simulink model "Model_14Bus_Microgrid_R2017b"  (R2017b)
settings: Solver=ode23tb  StartTime=0.0  StopTime=0.35  MaxStep=1e-2  RelTol=1e-3
InitFcn:
  | Set_parameters_R2018
StopFcn:
  | Save_Data;
  | Graphics;
values from neighbouring files (symbols this model uses):
  Clink = Ceq*2    (= 0.217013888889)    [Set_parameters_R2017b.m]    (also in Set_parameters_R2018.m)
  dis1 = 0.15    [Set_parameters_R2017b.m]    (also in Set_parameters_R2018.m)
  dis10 = 6    [Set_parameters_R2017b.m]    (also in Set_parameters_R2018.m)
  dis11 = 3    [Set_parameters_R2017b.m]    (also in Set_parameters_R2018.m)
  dis12 = 6    [Set_parameters_R2017b.m]    (also in Set_parameters_R2018.m)
  dis13 = 3    [Set_parameters_R2017b.m]    (also in Set_parameters_R2018.m)
  dis14 = 2    [Set_parameters_R2017b.m]    (also in Set_parameters_R2018.m)
  dis2 = 0.2    [Set_parameters_R2017b.m]    (also in Set_parameters_R2018.m)
  dis3 = 0.15    [Set_parameters_R2017b.m]    (also in Set_parameters_R2018.m)
  dis4 = 0.4    [Set_parameters_R2017b.m]    (also in Set_parameters_R2018.m)
  dis5 = 0.4    [Set_parameters_R2017b.m]    (also in Set_parameters_R2018.m)
  dis6 = 0.4    [Set_parameters_R2017b.m]    (also in Set_parameters_R2018.m)
  dis7 = 0.1    [Set_parameters_R2017b.m]    (also in Set_parameters_R2018.m)
  dis8 = 2    [Set_parameters_R2017b.m]    (also in Set_parameters_R2018.m)
  dis9 = 6    [Set_parameters_R2017b.m]    (also in Set_parameters_R2018.m)
  Fc = 33 * Fnom    (= 1980)    [Set_parameters_R2017b.m]    (also in Set_parameters_R2018.m)
  Fnom = 60    [Main_DC_MG.m]    (also in Set_parameters_R2017b.m; Set_parameters_R2018.m)
  Increment_MPPT = 0.01    [Set_parameters_R2017b.m]    (also in Set_parameters_R2018.m)
  Ki_Ireg = 20    [Set_parameters_R2017b.m]    (also in Set_parameters_R2018.m)
  Ki_VDCreg = 400    [Set_parameters_R2017b.m]    (also in Set_parameters_R2018.m)
  Kp_Ireg = 0.3    [Set_parameters_R2017b.m]    (also in Set_parameters_R2018.m)
  Kp_VDCreg = 2    [Set_parameters_R2017b.m]    (also in Set_parameters_R2018.m)
  LimitL_Ireg = -1.5    [Set_parameters_R2017b.m]    (also in Set_parameters_R2018.m)
  LimitL_VDCreg = -1.5    [Set_parameters_R2017b.m]    (also in Set_parameters_R2018.m)
  Limits_MPPT = [ 583 357 ]    [Set_parameters_R2017b.m]    (also in Set_parameters_R2018.m)
  LimitU_Ireg = 1.5    [Set_parameters_R2017b.m]    (also in Set_parameters_R2018.m)
  LimitU_VDCreg = 1.5    [Set_parameters_R2017b.m]    (also in Set_parameters_R2018.m)
  P_Load_2 = S_Load_2* PF_Load_2    (= 36000)    [Set_parameters_R2017b.m]    (also in Set_parameters_R2018.m)
  P_Load_3 = S_Load_3* PF_Load_3    (= 25500)    [Set_parameters_R2017b.m]    (also in Set_parameters_R2018.m)
  Pnom = 1e6    (= 1000000)    [Set_parameters_R2017b.m]    (also in Set_parameters_R2018.m)
  Pnom_T1 = 1.5e6    (= 1500000)    [Set_parameters_R2017b.m]    (also in Set_parameters_R2018.m)
  Pnom_T2 = 1.5e6    (= 1500000)    [Set_parameters_R2017b.m]    (also in Set_parameters_R2018.m)
  Pnom_T3 = 4e6    (= 4000000)    [Set_parameters_R2017b.m]    (also in Set_parameters_R2018.m)
  Pnom_xfo = Pnom    (= 1000000)    [Set_parameters_R2017b.m]    (also in Set_parameters_R2018.m)
  Ql_Load_2 = S_Load_2 * sin(acos(PF_Load_2))    [Set_parameters_R2017b.m]    (also in Set_parameters_R2018.m)
  Ql_Load_3 = S_Load_3 * sin(acos(PF_Load_3))    [Set_parameters_R2017b.m]    (also in Set_parameters_R2018.m)
  R_Load_9 = (Vnom_prim * 1.35)^2 / P_Load_9    (= 1084.6153125)    [Set_parameters_R2017b.m]    (also in Set_parameters_R2018.m)
  R_Load_DC = Vnom_DC^2/ P_Load_DC    (= 45)    [Main_DC_MG.m]    (also in Set_parameters_R2017b.m; Set_parameters_R2018.m)
  Rl = 0.394    [Set_parameters_R2017b.m]    (also in Set_parameters_R2018.m)
  Rls = 0.198    [Set_parameters_R2017b.m]    (also in Set_parameters_R2018.m)
  Ts = Ts_Power    (= 5.05050505051e-06)    [Main_DC_MG.m]    (also in Set_parameters_R2017b.m; Set_parameters_R2018.m)
  Ts_Control = 10*Ts_Power    (= 5.05050505051e-05)    [Main_DC_MG.m]    (also in Set_parameters_R2017b.m; Set_parameters_R2018.m)
  Ts_Power = 1/(33*Fnom)/100    (= 5.05050505051e-06)    [Main_DC_MG.m]    (also in Set_parameters_R2017b.m; Set_parameters_R2018.m)
  V1_LL_T3 = 69e3    (= 69000)    [Set_parameters_R2017b.m]    (also in Set_parameters_R2018.m)
  Vf = 0    [Set_parameters_R2017b.m]    (also in Set_parameters_R2018.m)
  Vfd = 0    [Set_parameters_R2017b.m]    (also in Set_parameters_R2018.m)
  Vnom_DC = 300    [Main_DC_MG.m]    (also in Set_parameters_R2017b.m; Set_parameters_R2018.m)
  Vnom_dc = 480    [Set_parameters_R2017b.m]    (also in Set_parameters_R2018.m)
  Vnom_Diesel = 2.4e3    (= 2400)    [Set_parameters_R2017b.m]    (also in Set_parameters_R2018.m)
  Vnom_prim = 13.8e3    (= 13800)    [Set_parameters_R2017b.m]    (also in Set_parameters_R2018.m)
  Vnom_sec = 220    [Set_parameters_R2017b.m]    (also in Set_parameters_R2018.m)
  Vnom_ter_AC_DC = 150    [Set_parameters_R2017b.m]    (also in Set_parameters_R2018.m)
  Xl = 0.1168    [Set_parameters_R2017b.m]    (also in Set_parameters_R2018.m)
  Xls = 0.1089    [Set_parameters_R2017b.m]    (also in Set_parameters_R2018.m)
undefined symbols (not defined in the file or in its folder): D1, Delta, Hydride, Ion, Lithium, max_min, Metal, Nickel, RL, RLff, sigbuilder_block
libraries: powerlib x202, powerlib_meascontrol x152, simulink x14, powerlib_extras x14, electricdrivelib x4, re_lib x2
(part 4 of 10)

== system Model_14Bus_Microgrid_R2017b/Bus_AC//DC4 ==
  note: C
  note: B
  note: A
  note: C
  note: Linea - Neutro
  note: B
  note: A
  note: C
  note: B
  note: A
  Conv pu1 : Gain  Gain=sqrt (3) /Vnom_ter_AC_DC  SaturateOnIntegerOverflow=on  OutDataTypeStr=Inherit: Same as input  ParamDataTypeStr=Inherit: Same as input
  Conv pu2 : Gain  Gain=sqrt (3) /Vnom_ter_AC_DC  SaturateOnIntegerOverflow=on  OutDataTypeStr=Inherit: Same as input  ParamDataTypeStr=Inherit: Same as input
  Measurement1 : Scope  NumInputPorts=4
  PLL : Subsystem
  PLL (3ph) : powerlib_meascontrol/PLL/PLL (3ph)  Fmin=45  Par_Init=[0, 60]  ParK=[180, 3200, 1]  TcD=1e-4  MaxRateChangeFreq=12  FilterCutOffFreq=25  Ts=0  AGC=on
      settings: SourceProductName=Simscape Electrical
  Power Factor Block1 : Subsystem  mask(Power Factor Block){Freq=Fnom, Vinit=[0, 0], Iinit=[0, 0], Ts=0}
      mask prompts: Freq "Fundamental frequency (Hz):"; Vinit "Voltage initial input [ Mag, Phase (degrees) ]:"; Iinit "Current initial input [ Mag, Phase (degrees) ]:"; Ts "Sample time:"
      mask help:
      | Power Factor Block developed by Dr Rodney Tan
      | Version 1.01 (Aug 2016)
      |
      | Compute power factor and phase angle of AC circuit voltage-current pair at fundamental frequency.
      |
      | The computation is based on Power block and Complex number function block.
      |
      | For the first cycle of simulation, the outputs are held constant to the powers computed for the Voltage initial input and Current initial input parameters.
      mask Help:
      | <b>Fundamental Frequency (Hz)</b>
      | Specify the measurement fundamental frequency, in hertz, of the input signal.
      | 
      | <b>Voltage initial input [ Mag, Phase (degrees) ]</b>
      | Specify the voltage initial magnitude and phase to set a constant output for the first cycle of simulation.
      | 
      | <b>Current initial input [ Mag, Phase (degrees) ]</b>
      | Specify the current initial magnitude and phase to set a constant output for the first cycle of simulation.
      | 
      | <b>Sample Time</b>
      | Specify the sample time of the block, in seconds. Set to 0 to implement a continuous block.
      mask TypeOptions Freq: Power/Freq
      mask TypeOptions Vinit: Power/Vinit
      mask TypeOptions Iinit: Power/Iinit
      mask TypeOptions Ts: Power/Ts
  Power Factor1 : Display
  Scope : Scope
  Scope1 : Scope
  Scope2 : Scope
  THD : powerlib_meascontrol/Measurements/THD  Freq=60  Ts=Ts_Power
      settings: SourceProductName=Simscape Electrical
  THD (% and signal) : Scope  NumInputPorts=2
  THD (%) : Display
      settings: Format=bank
  Terminator : Terminator
  Vabc pu1 : Scope
  frecuency (Hz) : Display
  to % : Gain  Gain=100  SampleTime=Ts_Power
  ángulo de V (%)1 : Display
      settings: Format=bank
  wires:
  [Iabc_B1_busDC1] -> Power Factor Block1/2(Iabc)
  THD/1 -> to %/1
  to %/1 -> THD (%)/1, THD (% and signal)/2  "THD (%)"
  Power Factor Block1/4(Iabc y Iabc (rms)) -> Measurement1/4
  Power Factor Block1/1(Pabc) -> Measurement1/1
  Conv pu1/1 -> Vabc pu1/1
  Power Factor Block1/5("PFabc ") -> Scope1/1, Power Factor1/1
  Power Factor Block1/2(Qabc) -> Measurement1/2
  Power Factor Block1/3(Vabc y Vabc (rms)) -> Conv pu1/1, Measurement1/3
  PLL/1(delta_abc) -> Scope/1, ángulo de V (%)1/1
  Conv pu2/1 -> PLL/1(Vabc_LN_pu)
  PLL (3ph)/2 -> Terminator/1
  [Vabc_B1_busDC1] -> PLL (3ph)/1, Conv pu2/1, THD/1, THD (% and signal)/1, Power Factor Block1/1(Vabc)  "Vabc"
  PLL (3ph)/1 -> Scope2/1, frecuency (Hz)/1

== system Model_14Bus_Microgrid_R2017b/Bus_AC//DC5 ==
  note: C
  note: B
  note: A
  note: C
  note: Linea - Neutro
  note: B
  note: A
  note: B
  note: C
  note: A
  Conv pu1 : Gain  Gain=sqrt (3) /Vnom_ter_AC_DC  SaturateOnIntegerOverflow=on  OutDataTypeStr=Inherit: Same as input  ParamDataTypeStr=Inherit: Same as input
  Conv pu2 : Gain  Gain=sqrt (3) /Vnom_ter_AC_DC  SaturateOnIntegerOverflow=on  OutDataTypeStr=Inherit: Same as input  ParamDataTypeStr=Inherit: Same as input
  Measurement1 : Scope  NumInputPorts=4
  PLL : Subsystem
  PLL (3ph) : powerlib_meascontrol/PLL/PLL (3ph)  Fmin=45  Par_Init=[0, 60]  ParK=[180, 3200, 1]  TcD=1e-4  MaxRateChangeFreq=12  FilterCutOffFreq=25  Ts=0  AGC=on
      settings: SourceProductName=Simscape Electrical
  Power Factor Block1 : Subsystem  mask(Power Factor Block){Freq=Fnom, Vinit=[0, 0], Iinit=[0, 0], Ts=0}
      mask prompts: Freq "Fundamental frequency (Hz):"; Vinit "Voltage initial input [ Mag, Phase (degrees) ]:"; Iinit "Current initial input [ Mag, Phase (degrees) ]:"; Ts "Sample time:"
      mask help:
      | Power Factor Block developed by Dr Rodney Tan
      | Version 1.01 (Aug 2016)
      |
      | Compute power factor and phase angle of AC circuit voltage-current pair at fundamental frequency.
      |
      | The computation is based on Power block and Complex number function block.
      |
      | For the first cycle of simulation, the outputs are held constant to the powers computed for the Voltage initial input and Current initial input parameters.
      mask Help:
      | <b>Fundamental Frequency (Hz)</b>
      | Specify the measurement fundamental frequency, in hertz, of the input signal.
      | 
      | <b>Voltage initial input [ Mag, Phase (degrees) ]</b>
      | Specify the voltage initial magnitude and phase to set a constant output for the first cycle of simulation.
      | 
      | <b>Current initial input [ Mag, Phase (degrees) ]</b>
      | Specify the current initial magnitude and phase to set a constant output for the first cycle of simulation.
      | 
      | <b>Sample Time</b>
      | Specify the sample time of the block, in seconds. Set to 0 to implement a continuous block.
      mask TypeOptions Freq: Power/Freq
      mask TypeOptions Vinit: Power/Vinit
      mask TypeOptions Iinit: Power/Iinit
      mask TypeOptions Ts: Power/Ts
  Power Factor1 : Display
  Scope : Scope
  Scope1 : Scope
  Scope2 : Scope
  THD : powerlib_meascontrol/Measurements/THD  Freq=60  Ts=Ts_Power
      settings: SourceProductName=Simscape Electrical
  THD (% and signal) : Scope  NumInputPorts=2
  THD (%) : Display
      settings: Format=bank
  Terminator : Terminator
  Vabc pu1 : Scope
  frecuency (Hz) : Display
  to % : Gain  Gain=100  SampleTime=Ts_Power
  ángulo de V (%)1 : Display
      settings: Format=bank
  wires:
  [Iabc_B1_busDC2] -> Power Factor Block1/2(Iabc)
  THD/1 -> to %/1
  to %/1 -> THD (%)/1, THD (% and signal)/2  "THD (%)"
  Power Factor Block1/4(Iabc y Iabc (rms)) -> Measurement1/4
  Power Factor Block1/1(Pabc) -> Measurement1/1
  Conv pu1/1 -> Vabc pu1/1
  Power Factor Block1/5("PFabc ") -> Scope1/1, Power Factor1/1
  Power Factor Block1/2(Qabc) -> Measurement1/2
  Power Factor Block1/3(Vabc y Vabc (rms)) -> Conv pu1/1, Measurement1/3
  Conv pu2/1 -> PLL/1(Vabc_LN_pu)
  PLL/1(delta_abc) -> Scope/1, ángulo de V (%)1/1
  PLL (3ph)/2 -> Terminator/1
  [Vabc_B1_busDC2] -> Power Factor Block1/1(Vabc), PLL (3ph)/1, Conv pu2/1, THD/1, THD (% and signal)/1  "Vabc"
  PLL (3ph)/1 -> Scope2/1, frecuency (Hz)/1

== system Model_14Bus_Microgrid_R2017b/Bus_slack  ==
  note: C
  note: B
  note: A
  note: C
  note: Linea - Neutro
  note: B
  note: A
  note: A
  note: B
  note: C
  Conv pu1 : Gain  Gain=sqrt (3) /Vnom_prim  SaturateOnIntegerOverflow=on  OutDataTypeStr=Inherit: Same as input  ParamDataTypeStr=Inherit: Same as input
  Conv pu2 : Gain  Gain=sqrt (3) /Vnom_prim  SaturateOnIntegerOverflow=on  OutDataTypeStr=Inherit: Same as input  ParamDataTypeStr=Inherit: Same as input
  Measurement1 : Scope  NumInputPorts=4
  PLL : Subsystem
  PLL (3ph) : powerlib_meascontrol/PLL/PLL (3ph)  Fmin=45  Par_Init=[0, 60]  ParK=[180, 3200, 1]  TcD=1e-4  MaxRateChangeFreq=12  FilterCutOffFreq=25  Ts=0  AGC=on
      settings: SourceProductName=Simscape Electrical
  Power Factor Block1 : Subsystem  mask(Power Factor Block){Freq=Fnom, Vinit=[0, 0], Iinit=[0, 0], Ts=0}
      mask prompts: Freq "Fundamental frequency (Hz):"; Vinit "Voltage initial input [ Mag, Phase (degrees) ]:"; Iinit "Current initial input [ Mag, Phase (degrees) ]:"; Ts "Sample time:"
      mask help:
      | Power Factor Block developed by Dr Rodney Tan
      | Version 1.01 (Aug 2016)
      |
      | Compute power factor and phase angle of AC circuit voltage-current pair at fundamental frequency.
      |
      | The computation is based on Power block and Complex number function block.
      |
      | For the first cycle of simulation, the outputs are held constant to the powers computed for the Voltage initial input and Current initial input parameters.
      mask Help:
      | <b>Fundamental Frequency (Hz)</b>
      | Specify the measurement fundamental frequency, in hertz, of the input signal.
      | 
      | <b>Voltage initial input [ Mag, Phase (degrees) ]</b>
      | Specify the voltage initial magnitude and phase to set a constant output for the first cycle of simulation.
      | 
      | <b>Current initial input [ Mag, Phase (degrees) ]</b>
      | Specify the current initial magnitude and phase to set a constant output for the first cycle of simulation.
      | 
      | <b>Sample Time</b>
      | Specify the sample time of the block, in seconds. Set to 0 to implement a continuous block.
      mask TypeOptions Freq: Power/Freq
      mask TypeOptions Vinit: Power/Vinit
      mask TypeOptions Iinit: Power/Iinit
      mask TypeOptions Ts: Power/Ts
  Power Factor1 : Display
  Scope : Scope
  Scope2 : Scope
  THD : powerlib_meascontrol/Measurements/THD  Freq=60  Ts=Ts_Power
      settings: SourceProductName=Simscape Electrical
  THD (% and signal) : Scope  NumInputPorts=2
  THD (%) : Display
      settings: Format=bank
  Terminator : Terminator
  Vabc pu1 : Scope
  frecuency (Hz) : Display
  to % : Gain  Gain=100  SampleTime=Ts_Power
  ángulo de V (%)1 : Display
      settings: Format=bank
  tag scope: PFabc_Bus13=global, THDv_abc_Bus13=global, delta_abc_Bus13=global
  wires:
  [Iabc_Sec] -> Power Factor Block1/2(Iabc)  "Signal Iabc"
  THD/1 -> to %/1
  Power Factor Block1/4(Iabc y Iabc (rms)) -> Measurement1/4
  Power Factor Block1/1(Pabc) -> Measurement1/1
  Conv pu1/1 -> Vabc pu1/1
  Power Factor Block1/2(Qabc) -> Measurement1/2
  Power Factor Block1/3(Vabc y Vabc (rms)) -> Conv pu1/1, Measurement1/3
  to %/1 -> [THDv_abc_Bus13], THD (%)/1, THD (% and signal)/2  "THD (%)"
  Power Factor Block1/5("PFabc ") -> [PFabc_Bus13], Power Factor1/1
  Conv pu2/1 -> PLL/1(Vabc_LN_pu)
  PLL/1(delta_abc) -> [delta_abc_Bus13], Scope/1, ángulo de V (%)1/1
  [Vabc_Sec] -> Power Factor Block1/1(Vabc), THD/1, THD (% and signal)/1, PLL (3ph)/1, Conv pu2/1  "Vabc"
  PLL (3ph)/2 -> Terminator/1
  PLL (3ph)/1 -> Scope2/1, frecuency (Hz)/1

== system Model_14Bus_Microgrid_R2017b/Control measurement ==
  note: VL-L rms
  Bus Creator : BusCreator  Inputs=4
  VL-L : Scope  NumInputPorts=2
  Vph_rms : Scope
  m1 : Scope
  measurement : Subsystem
  "                                          C" : PMIOPort  Side=Left
  "                                          B" : PMIOPort  Port=2  Side=Left
  "                                          A" : PMIOPort  Port=3  Side=Left
  "              Out1" : Outport
  wires:
  measurement/2(VL-L) -> VL-L/1, Bus Creator/2
  measurement/3(VL-L_rms) -> VL-L/2, Bus Creator/3
  measurement/4(Vph_rms) -> Vph_rms/1, Bus Creator/4
  measurement/1(Vph) -> m1/1, Bus Creator/1
  Bus Creator/1 -> "              Out1"/1
  connections:
  "                                          A"/RConn1 -- measurement/LConn1
  "                                          B"/RConn1 -- measurement/LConn2
  "                                          C"/RConn1 -- measurement/LConn3

== system Model_14Bus_Microgrid_R2017b/Control measurement2 ==
  note: VL-L rms_3
  Bus Creator : BusCreator  Inputs=4
  VL-L_3 : Scope  NumInputPorts=2
  Vph_rms_3 : Scope
  m1_3 : Scope
  measurement2 : Subsystem
  "                                          C" : PMIOPort  Side=Left
  "                                          B" : PMIOPort  Port=2  Side=Left
  "                                          A" : PMIOPort  Port=3  Side=Left
  "              Out1" : Outport
  wires:
  measurement2/2(VL-L) -> VL-L_3/1, Bus Creator/2
  measurement2/3(VL-L_rms) -> VL-L_3/2, Bus Creator/3
  measurement2/4(Vph_rms) -> Vph_rms_3/1, Bus Creator/4
  measurement2/1(Vph) -> m1_3/1, Bus Creator/1
  Bus Creator/1 -> "              Out1"/1
  connections:
  "                                          A"/RConn1 -- measurement2/LConn1
  "                                          B"/RConn1 -- measurement2/LConn2
  "                                          C"/RConn1 -- measurement2/LConn3

== system Model_14Bus_Microgrid_R2017b/DATA  ADQUISITION ==
  note: Transformer (T1)
  note: Paper: "Hybrid AC/DC Microgrid test system simulation: Grid-connected mode"
  Delta_abc : Subsystem
  PF_abc : Subsystem
  P_abc : Subsystem
  Power_Losses_abc : Subsystem
  Q_abc : Subsystem
  RMS1 : powerlib_meascontrol/Measurements/RMS  TrueRMS=on  Freq=60  RMSInit=0  Ts=0
      settings: SourceProductName=Simscape Electrical
  RMS2 : powerlib_meascontrol/Measurements/RMS  TrueRMS=on  Freq=60  RMSInit=0  Ts=0
      settings: SourceProductName=Simscape Electrical
  THDv_abc : Subsystem
  VoltageLL_pu_abc : Subsystem
  scope 11 : Scope
  scope 12 : Scope
  wires:
  [Vabc_Sec_pu] -> RMS1/1
  RMS1/1 -> scope 11/1
  RMS2/1 -> scope 12/1
  [Vabc_Prim_pu] -> RMS2/1  "Signal Vabc"

== system Model_14Bus_Microgrid_R2017b/Diesel_ 3MVA ==
  note: Diesel generator 2
  2.4kV  50MVA : powerlib/Elements/Three-Phase Series RLC Branch  LConnTagsString=A|B|C  RConnTagsString=A|B|C  BranchType=RL  Resistance=2.4e3^2/50e6/10  Inductance=2.4e3^2/50e6/(2*pi*60)  Capacitance=1.0  Measurements=None
      settings: SourceProductName=Simscape Electrical
  Ground1 : powerlib/Elements/Ground  LConnTagsString=a
      settings: SourceProductName=Simscape Electrical
  Programmable Voltage Source1 : powerlib/Electrical Sources/Three-Phase Programmable Voltage Source  PositiveSequence="[Vnom_Diesel*0.9848 -60  Fnom]"  VariationEntity=None  VariationType=Table of time-amplitude pairs  VariationTypeAlt=Step  VariationStep=-0.3  VariationRate=0.5  VariationMagnitude=0.4  VariationFrequency=2  VariationTiming=[0.1 1.2]  VariationPhaseA=off  Amplitudes=[1]  TimeValues=[0]  HarmonicGeneration=off  HarmonicA=[3 0.2 -25 0]  HarmonicB="[2 0.15  35 2]"  Timing="[0.1  0.6]"  BusType=PV  Pref=Pgen_Diesel  Qref=0  Qmin=-inf  Qmax=inf
      settings: SourceProductName=Simscape Electrical
  a1 : PMIOPort  Tag=PMCPort  Side=Left
  b1 : PMIOPort  Tag=PMCPort  Port=2  Side=Left
  c1 : PMIOPort  Tag=PMCPort  Port=3  Side=Left
  connections:
  Programmable Voltage Source1/RConn3 -- 2.4kV  50MVA/LConn3
  Ground1/LConn1 -- Programmable Voltage Source1/LConn1
  Programmable Voltage Source1/RConn2 -- 2.4kV  50MVA/LConn2
  2.4kV  50MVA/LConn1 -- Programmable Voltage Source1/RConn1
  b1/RConn1 -- 2.4kV  50MVA/RConn2
  a1/RConn1 -- 2.4kV  50MVA/RConn1
  c1/RConn1 -- 2.4kV  50MVA/RConn3

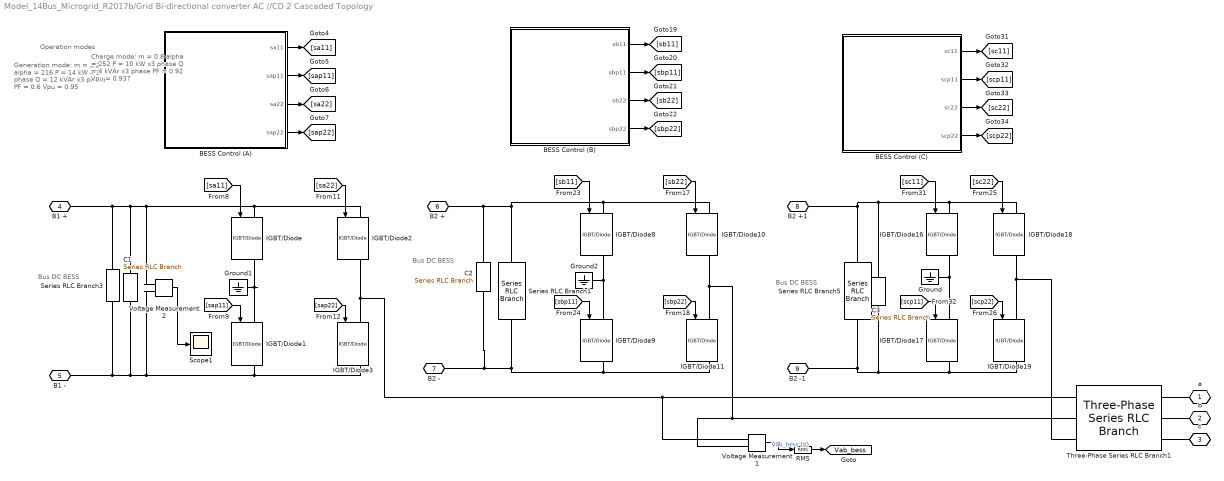
== system Model_14Bus_Microgrid_R2017b/Grid Bi-directional converter AC //CD 2 Cascaded Topology ==
  note: Operation modes
  note: Generation mode:
      |
      | m = 1.2
      | alpha = 216
      |
      | P = 14 kW x 3 phase
      | Q = 12 kVAr x3 phase
      | PF = 0.6
      | Vpu = 0.95
  note: Bus DC BESS
  note: Bus DC BESS
  note: Bus DC BESS
  note: Charge mode:
      |
      | m = 0.8
      | alpha = 252
      |
      | P = 10 kW x3 phase
      | Q = 4 kVAr x3 phase
      | PF = 0.92
      | Vpu = 0.937
  BESS Control (A) : Subsystem
      mask Display: image('Icons\FPGA.png');
  BESS Control (B) : Subsystem
      mask Display: image('Icons\FPGA.png');
  BESS Control (C) : Subsystem
      mask Display: image('Icons\FPGA.png');
  C1 : powerlib/Elements/Series RLC Branch  LConnTagsString=__new0  RConnTagsString=__new0  BranchType=C  Resistance=22.5  Inductance=1e-3  SetiL0=off  InitialCurrent=0  Capacitance=10e-3  Setx0=off  InitialVoltage=0  Measurements=None
      settings: SourceProductName=Simscape Electrical
  C2 : powerlib/Elements/Series RLC Branch  LConnTagsString=__new0  RConnTagsString=__new0  BranchType=C  Resistance=22.5  Inductance=1e-3  SetiL0=off  InitialCurrent=0  Capacitance=10e-3  Setx0=off  InitialVoltage=0  Measurements=None
      settings: SourceProductName=Simscape Electrical
  C3 : powerlib/Elements/Series RLC Branch  LConnTagsString=__new0  RConnTagsString=__new0  BranchType=C  Resistance=22.5  Inductance=1e-3  SetiL0=off  InitialCurrent=0  Capacitance=10e-3  Setx0=off  InitialVoltage=0  Measurements=None
      settings: SourceProductName=Simscape Electrical
  Ground : powerlib/Elements/Ground  LConnTagsString=a
      settings: SourceProductName=Simscape Electrical
  Ground1 : powerlib/Elements/Ground  LConnTagsString=a
      settings: SourceProductName=Simscape Electrical
  Ground2 : powerlib/Elements/Ground  LConnTagsString=a
      settings: SourceProductName=Simscape Electrical
  IGBT/Diode{,1..3,8..11,16..19} (12 alike) : powerlib/Power Electronics/IGBT//Diode  Ron=1e-3  Rs=1e5  Cs=inf  Measurements=on
      settings: SourceProductName=Simscape Electrical
  RMS : powerlib_meascontrol/Measurements/RMS  TrueRMS=off  Freq=60  RMSInit=1  Ts=0
      settings: SourceProductName=Simscape Electrical
  Scope1 : Scope
  Series RLC Branch1 : powerlib/Elements/Series RLC Branch  LConnTagsString=__new0  RConnTagsString=__new0  BranchType=R  Resistance=1e9  Inductance=1e-3  SetiL0=off  InitialCurrent=0  Capacitance=1e-6  Setx0=off  InitialVoltage=0  Measurements=None
      settings: SourceProductName=Simscape Electrical
  Series RLC Branch3 : powerlib/Elements/Series RLC Branch  LConnTagsString=__new0  RConnTagsString=__new0  BranchType=R  Resistance=1e9  Inductance=1e-3  SetiL0=off  InitialCurrent=0  Capacitance=1e-6  Setx0=off  InitialVoltage=0  Measurements=None
      settings: SourceProductName=Simscape Electrical
  Series RLC Branch5 : powerlib/Elements/Series RLC Branch  LConnTagsString=__new0  RConnTagsString=__new0  BranchType=R  Resistance=1e9  Inductance=1e-3  SetiL0=off  InitialCurrent=0  Capacitance=1e-6  Setx0=off  InitialVoltage=0  Measurements=None
      settings: SourceProductName=Simscape Electrical
  Three-Phase Series RLC Branch1 : powerlib/Elements/Three-Phase Series RLC Branch  LConnTagsString=A|B|C  RConnTagsString=A|B|C  BranchType=RL  Resistance=1  Inductance=1.2e-2  Capacitance=15.5e-5  Measurements=None
      settings: SourceProductName=Simscape Electrical
  Voltage Measurement1 : powerlib/Measurements/Voltage Measurement  PhasorSimulation=off  OutputType=Complex  PSBequivalent=0
      settings: SourceProductName=Simscape Electrical
  Voltage Measurement2 : powerlib/Measurements/Voltage Measurement  PhasorSimulation=off  OutputType=Complex  PSBequivalent=0
      settings: SourceProductName=Simscape Electrical
  "a " : PMIOPort  Tag=PMCPort  Side=Left
  b : PMIOPort  Tag=PMCPort  Port=2  Side=Left
  c : PMIOPort  Tag=PMCPort  Port=3  Side=Left
  B1 + : PMIOPort  Port=4  Side=Right
  B1 - : PMIOPort  Port=5  Side=Right
  B2 + : PMIOPort  Port=6  Side=Right
  B2 - : PMIOPort  Port=7  Side=Right
  B2 +1 : PMIOPort  Port=8  Side=Right
  B2 -1 : PMIOPort  Port=9  Side=Right
  tag scope: Vab_bess=global
  wires:
  [sa11] -> IGBT/Diode/1
  [sap11] -> IGBT/Diode1/1
  [sa22] -> IGBT/Diode2/1
  [sap22] -> IGBT/Diode3/1
  [sb11] -> IGBT/Diode8/1
  [sbp11] -> IGBT/Diode9/1
  [sb22] -> IGBT/Diode10/1
  [sbp22] -> IGBT/Diode11/1
  [sc11] -> IGBT/Diode16/1
  [scp11] -> IGBT/Diode17/1
  [sc22] -> IGBT/Diode18/1
  [scp22] -> IGBT/Diode19/1
  Voltage Measurement1/1 -> RMS/1  "Vab_bess (V)"
  RMS/1 -> [Vab_bess]
  Voltage Measurement2/1 -> Scope1/1
  BESS Control (A)/1(sa11) -> [sa11]
  BESS Control (A)/2(sap11) -> [sap11]
  BESS Control (A)/3(sa22) -> [sa22]
  BESS Control (A)/4(sap22) -> [sap22]
  BESS Control (B)/1(sb11) -> [sb11]
  BESS Control (B)/2(sbp11) -> [sbp11]
  BESS Control (B)/3(sb22) -> [sb22]
  BESS Control (B)/4(sbp22) -> [sbp22]
  BESS Control (C)/1(sc11) -> [sc11]
  BESS Control (C)/2(scp11) -> [scp11]
  BESS Control (C)/3(sc22) -> [sc22]
  BESS Control (C)/4(scp22) -> [scp22]
  connections:
  IGBT/Diode1/RConn1 -- IGBT/Diode3/RConn1 -- C1/RConn1 -- Series RLC Branch3/RConn1 -- B1 -/RConn1 -- Voltage Measurement2/LConn2
  Series RLC Branch1/RConn1 -- C2/RConn1 -- B2 -/RConn1 -- IGBT/Diode9/RConn1 -- IGBT/Diode11/RConn1
  IGBT/Diode11/LConn1 -- Voltage Measurement1/LConn2 -- Three-Phase Series RLC Branch1/LConn2 -- IGBT/Diode10/RConn1
  Series RLC Branch5/RConn1 -- B2 -1/RConn1 -- C3/RConn1 -- IGBT/Diode19/RConn1 -- IGBT/Diode17/RConn1
  IGBT/Diode19/LConn1 -- Three-Phase Series RLC Branch1/LConn3 -- IGBT/Diode18/RConn1
  IGBT/Diode/LConn1 -- IGBT/Diode2/LConn1 -- Voltage Measurement2/LConn1 -- C1/LConn1 -- B1 +/RConn1 -- Series RLC Branch3/LConn1
  Voltage Measurement1/LConn1 -- IGBT/Diode2/RConn1 -- IGBT/Diode3/LConn1 -- Three-Phase Series RLC Branch1/LConn1
  IGBT/Diode8/LConn1 -- C2/LConn1 -- B2 +/RConn1 -- Series RLC Branch1/LConn1 -- IGBT/Diode10/LConn1
  IGBT/Diode16/LConn1 -- C3/LConn1 -- Series RLC Branch5/LConn1 -- B2 +1/RConn1 -- IGBT/Diode18/LConn1
  IGBT/Diode1/LConn1 -- Ground1/LConn1 -- IGBT/Diode/RConn1
  IGBT/Diode9/LConn1 -- Ground2/LConn1 -- IGBT/Diode8/RConn1
  IGBT/Diode16/RConn1 -- Ground/LConn1 -- IGBT/Diode17/LConn1
  "a "/RConn1 -- Three-Phase Series RLC Branch1/RConn1
  b/RConn1 -- Three-Phase Series RLC Branch1/RConn2
  c/RConn1 -- Three-Phase Series RLC Branch1/RConn3

== system Model_14Bus_Microgrid_R2017b/Grid Bi-directional Converter 1.1 300 (DC) // 150 V (AC) P_nom 3kW ==
  note: Bus DC
  note: Bus AC
  note: Inverter mode:
      |
      | m = 1.2
      | alpha = 0
      |
      | P = 1 kW x 3 phase
      | Q = 1 kVAr x3 phase
      | PF = 0.6
      | Vpu = 0.95
  note: Operation modes
  note: Rectif mode:
      |
      | m = 1
      | alpha = 228
      |
      | P = 975 kVA (DC)
  Means : Inport
  C1 : powerlib/Elements/Series RLC Branch  LConnTagsString=__new0  RConnTagsString=__new0  BranchType=C  Resistance=22.5  Inductance=1e-3  SetiL0=off  InitialCurrent=0  Capacitance=1200e-6  Setx0=off  InitialVoltage=150  Measurements=None
      settings: SourceProductName=Simscape Electrical
  Control of Inverter : Subsystem
      mask Display: image('Icons\FPGA.png');
  Ground1 : powerlib/Elements/Ground  LConnTagsString=a
      settings: SourceProductName=Simscape Electrical
  Scope : Scope
  Three-Phase Parallel RLC Branch1 : powerlib/Elements/Three-Phase Parallel RLC Branch  LConnTagsString=A|B|C  RConnTagsString=A|B|C  BranchType=C  Resistance=1  Inductance=1e-3  Capacitance=2.65e-6  Measurements=None
      settings: SourceProductName=Simscape Electrical  SourceProductBaseCode=PS
  Three-Phase Series RLC Branch1 : powerlib/Elements/Three-Phase Series RLC Branch  LConnTagsString=A|B|C  RConnTagsString=A|B|C  BranchType=RL  Resistance=2  Inductance=1e-2  Capacitance=15.5e-5  Measurements=None
      settings: SourceProductName=Simscape Electrical
  Universal Bridge1 : powerlib/Power Electronics/Universal Bridge  Arms=3  SnubberResistance=1e5  SnubberCapacitance=inf  Device=MOSFET / Diodes  Ron=1e-3  Lon=0  ForwardVoltages="[  0  0  ]"  ForwardVoltage=0  GTOparameters=[ 10e-6 , 20e-6 ]  IGBTparameters=[ 1e-6 , 2e-6 ]  Measurements=None  Measurements_2=None  converterType=Rectifier
      settings: SourceProductName=Simscape Electrical
  "a " : PMIOPort  Tag=PMCPort  Side=Left
  b : PMIOPort  Tag=PMCPort  Port=2  Side=Left
  c : PMIOPort  Tag=PMCPort  Port=3  Side=Left
  B1 + : PMIOPort  Port=4  Side=Right
  B1 - : PMIOPort  Port=5  Side=Right
  tag scope: Pulse=global
  wires:
  Control of Inverter/1(Pulses) -> Scope/1, [Pulse]
  [Pulse] -> Universal Bridge1/1
  Means/1 -> Control of Inverter/1(Means)
  connections:
  Three-Phase Series RLC Branch1/RConn1 -- Three-Phase Parallel RLC Branch1/LConn1 -- "a "/RConn1
  Three-Phase Parallel RLC Branch1/LConn2 -- Three-Phase Series RLC Branch1/RConn2 -- b/RConn1
  Three-Phase Parallel RLC Branch1/LConn3 -- Three-Phase Series RLC Branch1/RConn3 -- c/RConn1
  Ground1/LConn1 -- Three-Phase Parallel RLC Branch1/RConn3 -- Three-Phase Parallel RLC Branch1/RConn1 -- Three-Phase Parallel RLC Branch1/RConn2
  Universal Bridge1/LConn3 -- Three-Phase Series RLC Branch1/LConn3
  Three-Phase Series RLC Branch1/LConn2 -- Universal Bridge1/LConn2
  Universal Bridge1/LConn1 -- Three-Phase Series RLC Branch1/LConn1
  B1 +/RConn1 -- C1/LConn1 -- Universal Bridge1/RConn1
  B1 -/RConn1 -- C1/RConn1 -- Universal Bridge1/RConn2

== system Model_14Bus_Microgrid_R2017b/Grid Bi-directional Converter 1.2 300 (DC) // 150 V (AC) P_nom 3kW ==
  note: DC Bus
  note: AC Bus
  note: Inverter mode:
      |
      | m = 1.2
      | alpha = 0
      |
      | P = 1 kW x 3 phase
      | Q = 1 kVAr x3 phase
      | PF = 0.6
      | Vpu = 0.95
  note: Rectif mode:
      |
      | NO WORK
  Means2 : Inport
  C1 : powerlib/Elements/Series RLC Branch  LConnTagsString=__new0  RConnTagsString=__new0  BranchType=C  Resistance=22.5  Inductance=1e-3  SetiL0=off  InitialCurrent=0  Capacitance=1200e-6  Setx0=off  InitialVoltage=150  Measurements=None
      settings: SourceProductName=Simscape Electrical
  Control of Inverter : Subsystem
      mask Display: image('Icons\FPGA.png');
  Ground1 : powerlib/Elements/Ground  LConnTagsString=a
      settings: SourceProductName=Simscape Electrical
  Scope : Scope
  Three-Phase Parallel RLC Branch2 : powerlib/Elements/Three-Phase Parallel RLC Branch  LConnTagsString=A|B|C  RConnTagsString=A|B|C  BranchType=C  Resistance=1  Inductance=1e-3  Capacitance=2.65e-6  Measurements=None
      settings: SourceProductName=Simscape Electrical  SourceProductBaseCode=PS
  Three-Phase Series RLC Branch2 : powerlib/Elements/Three-Phase Series RLC Branch  LConnTagsString=A|B|C  RConnTagsString=A|B|C  BranchType=RL  Resistance=2  Inductance=1e-2  Capacitance=15.5e-5  Measurements=None
      settings: SourceProductName=Simscape Electrical
  Universal Bridge2 : powerlib/Power Electronics/Universal Bridge  Arms=3  SnubberResistance=1e5  SnubberCapacitance=inf  Device=MOSFET / Diodes  Ron=1e-3  Lon=0  ForwardVoltages="[  0  0  ]"  ForwardVoltage=0  GTOparameters=[ 10e-6 , 20e-6 ]  IGBTparameters=[ 1e-6 , 2e-6 ]  Measurements=None  Measurements_2=None  converterType=Rectifier
      settings: SourceProductName=Simscape Electrical
  "a " : PMIOPort  Tag=PMCPort  Side=Left
  b : PMIOPort  Tag=PMCPort  Port=2  Side=Left
  c : PMIOPort  Tag=PMCPort  Port=3  Side=Left
  B1 + : PMIOPort  Port=4  Side=Right
  B1 - : PMIOPort  Port=5  Side=Right
  tag scope: Pulse2=global
  wires:
  Control of Inverter/1(Pulses) -> Scope/1, [Pulse2]
  Means2/1 -> Control of Inverter/1(Means2)
  [Pulse2] -> Universal Bridge2/1
  connections:
  Three-Phase Series RLC Branch2/RConn1 -- Three-Phase Parallel RLC Branch2/LConn1 -- "a "/RConn1
  Three-Phase Parallel RLC Branch2/LConn2 -- Three-Phase Series RLC Branch2/RConn2 -- b/RConn1
  Three-Phase Parallel RLC Branch2/LConn3 -- Three-Phase Series RLC Branch2/RConn3 -- c/RConn1
  Ground1/LConn1 -- Three-Phase Parallel RLC Branch2/RConn3 -- Three-Phase Parallel RLC Branch2/RConn1 -- Three-Phase Parallel RLC Branch2/RConn2
  Universal Bridge2/LConn3 -- Three-Phase Series RLC Branch2/LConn3
  Three-Phase Series RLC Branch2/LConn2 -- Universal Bridge2/LConn2
  Universal Bridge2/LConn1 -- Three-Phase Series RLC Branch2/LConn1
  Universal Bridge2/RConn1 -- B1 +/RConn1 -- C1/LConn1
  B1 -/RConn1 -- Universal Bridge2/RConn2 -- C1/RConn1

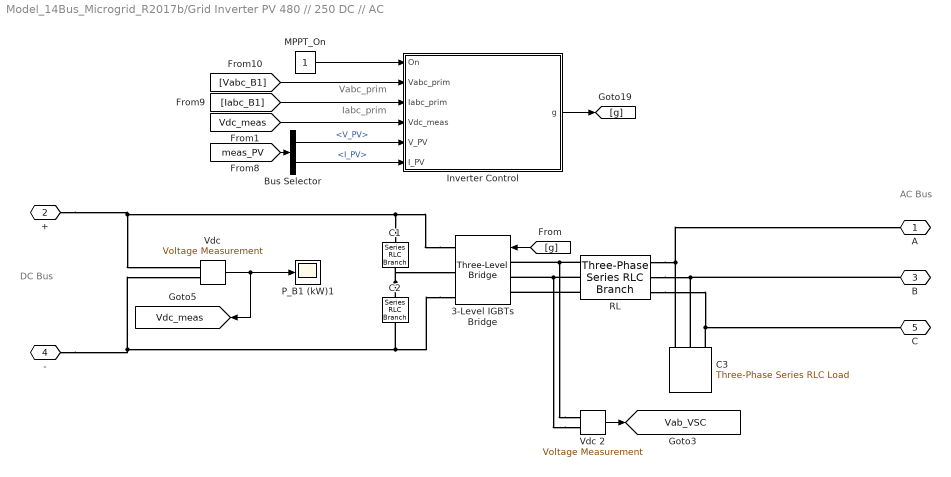
== system Model_14Bus_Microgrid_R2017b/Grid Inverter PV 480 // 250 DC // AC  ==
  note: Iabc_prim
  note: Vabc_prim
  note: AC Bus
  note: DC Bus
  3-Level IGBTs Bridge : powerlib/Power Electronics/Three-Level Bridge  Arms=3  SnubberResistance=Rs  SbubberCapacitance=Cs  Device=IGBT / Diodes  Ron=Ron  ForwardVoltages="[  Vfd  Vf ]"  Measurements=None
      settings: SourceProductName=Simscape Electrical  SourceProductBaseCode=PS
  Bus Selector : BusSelector  OutputSignals=V_PV,I_PV
  C1 : powerlib/Elements/Series RLC Branch  LConnTagsString=__new0  RConnTagsString=__new0  BranchType=C  Resistance=1.0  Inductance=1.0  SetiL0=off  InitialCurrent=0  Capacitance=Clink  Setx0=on  InitialVoltage=Vnom_dc/2  Measurements=None
      settings: SourceProductName=Simscape Electrical
  C2 : powerlib/Elements/Series RLC Branch  LConnTagsString=__new0  RConnTagsString=__new0  BranchType=C  Resistance=1.0  Inductance=1.0  SetiL0=off  InitialCurrent=0  Capacitance=Clink  Setx0=on  InitialVoltage=Vnom_dc/2  Measurements=None
      settings: SourceProductName=Simscape Electrical
  C3 : powerlib/Elements/Three-Phase Series RLC Load  LConnTagsString=A|B|C  Configuration=Delta  NominalVoltage=Vnom_sec  Vabc=[1e3 1e3 1e3]  Vabcp=[1e3 1e3 1e3]  NominalFrequency=Fnom  UnbalancedPower=off  ActivePower=Pc  InductivePower=0  CapacitivePower=Qc  Pabc=[10e3 9e3 11e3]  QLabc=[100 90 110]  QCabc=[100 90 110]  Pabcp=[10e3 9e3 11e3]  QLabcp=[100 90 110]  QCabcp=[100 90 110]  Measurements=None  LoadType=constant Z
      settings: SourceProductName=Simscape Electrical
  Inverter Control : Subsystem  mask(Inverter Control){Pnom=Pnom, Fnom=Fnom, Vnom_prim=Vnom_prim, Vnom_sec=Vnom_sec, Vnom_dc=Vnom_dc, Increment_MPPT=Increment_MPPT, Limits_MPPT=Limits_MPPT, Vdc_ref_Init=Vnom_dc, Kp_VDCreg=Kp_VDCreg, Ki_VDCreg=Ki_VDCreg, Kp_Ireg=Kp_Ireg, Ki_Ireg=Ki_Ireg, RLff=RLff, Fc=Fc, Ts_Control=Ts_Control, Ts_PWMgenerator=Ts_Power}
      mask prompts: Pnom "Power (VA)"; Fnom "Frequency (Hz)"; Vnom_prim "Primary voltage (Vrms LL)"; Vnom_sec "Secondary voltage (Vrms LL)"; Vnom_dc "DC voltage (V)"; Increment_MPPT "Output increment (V)"; Limits_MPPT "Output limits [ Upper  Lower ]"; Vdc_ref_Init "Output initial value (V)"; Kp_VDCreg "Proportional gain"; Ki_VDCreg "Integral gain"; Kp_Ireg "Proportional gain"; Ki_Ireg "Integral gain"; RLff "Feedforward Values [Rff Lff]"; Fc "Carrier frequency (Hz)"; Ts_Control "Control systems"; Ts_PWMgenerator "PWM generator"
      mask help:
      | The main components of the Inverter Control are:
      | 1. PLL & Measurements
      | 2. Maximum Power Point Tracker System (MPPT) using a Perturb & Observe algorithm
      | 3. DC Voltage Regulator
      | 4. Current Regulator
      | 5. PWM Modulator
      mask DialogControl Container4 Prompt: Nominal Values:
      mask DialogControl Container3 Prompt: MPPT Controller:
      mask DialogControl Container8 Prompt: Dc Voltage Regulator:
      mask DialogControl Container6 Prompt: Current Regulator:
      mask DialogControl Container9 Prompt: PWM Modulator:
      mask DialogControl SampleTimes Prompt: Sample Times:
      mask Display: image('Icons\FPGA.png');
  MPPT_On : Constant
  P_B1 (kW)1 : Scope
  RL : powerlib/Elements/Three-Phase Series RLC Branch  LConnTagsString=A|B|C  RConnTagsString=A|B|C  BranchType=RL  Resistance=RL(1)  Inductance=RL(2)  Capacitance=inf  Measurements=None
      settings: SourceProductName=Simscape Electrical
  "Vdc " : powerlib/Measurements/Voltage Measurement  Tag=PoWeRsYsTeMmEaSuReMeNt  PhasorSimulation=off  OutputType=Magnitude  PSBequivalent=0
      settings: SourceProductName=Simscape Electrical
  Vdc 2 : powerlib/Measurements/Voltage Measurement  Tag=PoWeRsYsTeMmEaSuReMeNt  PhasorSimulation=off  OutputType=Magnitude  PSBequivalent=0
      settings: SourceProductName=Simscape Electrical
  A : PMIOPort  Side=Right
  + : PMIOPort  Port=2  Side=Left
  B : PMIOPort  Port=3  Side=Right
  - : PMIOPort  Port=4  Side=Left
  C : PMIOPort  Port=5  Side=Right
  tag scope: Vab_VSC=global, Vdc_meas=global
  wires:
  Bus Selector/1 -> Inverter Control/5(V_PV)  "<V_PV>"
  [Vdc_meas] -> Inverter Control/4(Vdc_meas)
  [meas_PV] -> Bus Selector/1
  MPPT_On/1 -> Inverter Control/1(On)
  [Vabc_B1] -> Inverter Control/2(Vabc_prim)
  [Iabc_B1] -> Inverter Control/3(Iabc_prim)
  Bus Selector/2 -> Inverter Control/6(I_PV)  "<I_PV>"
  "Vdc "/1 -> [Vdc_meas], P_B1 (kW)1/1
  Vdc 2/1 -> [Vab_VSC]
  Inverter Control/1(g) -> [g]
  [g] -> 3-Level IGBTs Bridge/1
  connections:
  Vdc 2/LConn1 -- 3-Level IGBTs Bridge/LConn1 -- RL/LConn1
  Vdc 2/LConn2 -- 3-Level IGBTs Bridge/LConn2 -- RL/LConn2
  C3/LConn1 -- RL/RConn1 -- A/RConn1
  C3/LConn2 -- RL/RConn2 -- B/RConn1
  3-Level IGBTs Bridge/RConn3 -- -/RConn1 -- "Vdc "/LConn2 -- C2/RConn1
  C1/RConn1 -- C2/LConn1 -- 3-Level IGBTs Bridge/RConn2
  3-Level IGBTs Bridge/RConn1 -- C1/LConn1 -- "Vdc "/LConn1 -- +/RConn1
  RL/LConn3 -- 3-Level IGBTs Bridge/LConn3
  C3/LConn3 -- RL/RConn3 -- C/RConn1

== system Model_14Bus_Microgrid_R2017b/Load_1 ==
  note: C
  note: Linea - Neutro
  note: B
  note: A
  Conv pu1 : Gain  Gain=sqrt (3) /Vnom_sec  SaturateOnIntegerOverflow=on  OutDataTypeStr=Inherit: Same as input  ParamDataTypeStr=Inherit: Same as input
  Measurement1 : Scope  NumInputPorts=4
  Power Factor Block1 : Subsystem  mask(Power Factor Block){Freq=Fnom, Vinit=[0, 0], Iinit=[0, 0], Ts=0}
      mask prompts: Freq "Fundamental frequency (Hz):"; Vinit "Voltage initial input [ Mag, Phase (degrees) ]:"; Iinit "Current initial input [ Mag, Phase (degrees) ]:"; Ts "Sample time:"
      mask help:
      | Power Factor Block developed by Dr Rodney Tan
      | Version 1.01 (Aug 2016)
      |
      | Compute power factor and phase angle of AC circuit voltage-current pair at fundamental frequency.
      |
      | The computation is based on Power block and Complex number function block.
      |
      | For the first cycle of simulation, the outputs are held constant to the powers computed for the Voltage initial input and Current initial input parameters.
      mask Help:
      | <b>Fundamental Frequency (Hz)</b>
      | Specify the measurement fundamental frequency, in hertz, of the input signal.
      | 
      | <b>Voltage initial input [ Mag, Phase (degrees) ]</b>
      | Specify the voltage initial magnitude and phase to set a constant output for the first cycle of simulation.
      | 
      | <b>Current initial input [ Mag, Phase (degrees) ]</b>
      | Specify the current initial magnitude and phase to set a constant output for the first cycle of simulation.
      | 
      | <b>Sample Time</b>
      | Specify the sample time of the block, in seconds. Set to 0 to implement a continuous block.
      mask TypeOptions Freq: Power/Freq
      mask TypeOptions Vinit: Power/Vinit
      mask TypeOptions Iinit: Power/Iinit
      mask TypeOptions Ts: Power/Ts
  Power Factor1 : Display
  Vabc pu1 : Scope
  wires:
  [Iabc_load_1] -> Power Factor Block1/2(Iabc)
  [Vabc_load_1] -> Power Factor Block1/1(Vabc)
  Power Factor Block1/4(Iabc y Iabc (rms)) -> Measurement1/4
  Power Factor Block1/1(Pabc) -> Measurement1/1
  Conv pu1/1 -> Vabc pu1/1
  Power Factor Block1/5("PFabc ") -> Power Factor1/1
  Power Factor Block1/2(Qabc) -> Measurement1/2
  Power Factor Block1/3(Vabc y Vabc (rms)) -> Conv pu1/1, Measurement1/3

== system Model_14Bus_Microgrid_R2017b/Load_2 ==
  note: C
  note: B
  note: A
  note: C
  note: Linea - Neutro
  note: B
  note: A
  Conv pu1 : Gain  Gain=sqrt (3) /Vnom_sec  SaturateOnIntegerOverflow=on  OutDataTypeStr=Inherit: Same as input  ParamDataTypeStr=Inherit: Same as input
  Measurement1 : Scope  NumInputPorts=4
  Power Factor Block1 : Subsystem  mask(Power Factor Block){Freq=Fnom, Vinit=[0, 0], Iinit=[0, 0], Ts=0}
      mask prompts: Freq "Fundamental frequency (Hz):"; Vinit "Voltage initial input [ Mag, Phase (degrees) ]:"; Iinit "Current initial input [ Mag, Phase (degrees) ]:"; Ts "Sample time:"
      mask help:
      | Power Factor Block developed by Dr Rodney Tan
      | Version 1.01 (Aug 2016)
      |
      | Compute power factor and phase angle of AC circuit voltage-current pair at fundamental frequency.
      |
      | The computation is based on Power block and Complex number function block.
      |
      | For the first cycle of simulation, the outputs are held constant to the powers computed for the Voltage initial input and Current initial input parameters.
      mask Help:
      | <b>Fundamental Frequency (Hz)</b>
      | Specify the measurement fundamental frequency, in hertz, of the input signal.
      | 
      | <b>Voltage initial input [ Mag, Phase (degrees) ]</b>
      | Specify the voltage initial magnitude and phase to set a constant output for the first cycle of simulation.
      | 
      | <b>Current initial input [ Mag, Phase (degrees) ]</b>
      | Specify the current initial magnitude and phase to set a constant output for the first cycle of simulation.
      | 
      | <b>Sample Time</b>
      | Specify the sample time of the block, in seconds. Set to 0 to implement a continuous block.
      mask TypeOptions Freq: Power/Freq
      mask TypeOptions Vinit: Power/Vinit
      mask TypeOptions Iinit: Power/Iinit
      mask TypeOptions Ts: Power/Ts
  Power Factor1 : Display
  THD : powerlib_meascontrol/Measurements/THD  Freq=60  Ts=Ts_Power
      settings: SourceProductName=Simscape Electrical
  THD (% and signal) : Scope  NumInputPorts=2
  THD (%) : Display
      settings: Format=bank
  Vabc pu1 : Scope
  to % : Gain  Gain=100  SampleTime=Ts_Power
  wires:
  [Iabc_load_2] -> Power Factor Block1/2(Iabc)
  [Vabc_load_2] -> Power Factor Block1/1(Vabc), THD/1, THD (% and signal)/1  "Signal Vabc"
  THD/1 -> to %/1
  to %/1 -> THD (%)/1, THD (% and signal)/2  "THD (%)"
  Power Factor Block1/4(Iabc y Iabc (rms)) -> Measurement1/4
  Power Factor Block1/1(Pabc) -> Measurement1/1
  Conv pu1/1 -> Vabc pu1/1
  Power Factor Block1/5("PFabc ") -> Power Factor1/1
  Power Factor Block1/2(Qabc) -> Measurement1/2
  Power Factor Block1/3(Vabc y Vabc (rms)) -> Conv pu1/1, Measurement1/3

== system Model_14Bus_Microgrid_R2017b/Load_3 ==
  note: C
  note: B
  note: A
  note: C
  note: Linea - Neutro
  note: B
  note: A
  Conv pu1 : Gain  Gain=sqrt (3) /Vnom_prim  SaturateOnIntegerOverflow=on  OutDataTypeStr=Inherit: Same as input  ParamDataTypeStr=Inherit: Same as input
  Measurement1 : Scope  NumInputPorts=4
  Power Factor Block1 : Subsystem  mask(Power Factor Block){Freq=Fnom, Vinit=[0, 0], Iinit=[0, 0], Ts=0}
      mask prompts: Freq "Fundamental frequency (Hz):"; Vinit "Voltage initial input [ Mag, Phase (degrees) ]:"; Iinit "Current initial input [ Mag, Phase (degrees) ]:"; Ts "Sample time:"
      mask help:
      | Power Factor Block developed by Dr Rodney Tan
      | Version 1.01 (Aug 2016)
      |
      | Compute power factor and phase angle of AC circuit voltage-current pair at fundamental frequency.
      |
      | The computation is based on Power block and Complex number function block.
      |
      | For the first cycle of simulation, the outputs are held constant to the powers computed for the Voltage initial input and Current initial input parameters.
      mask Help:
      | <b>Fundamental Frequency (Hz)</b>
      | Specify the measurement fundamental frequency, in hertz, of the input signal.
      | 
      | <b>Voltage initial input [ Mag, Phase (degrees) ]</b>
      | Specify the voltage initial magnitude and phase to set a constant output for the first cycle of simulation.
      | 
      | <b>Current initial input [ Mag, Phase (degrees) ]</b>
      | Specify the current initial magnitude and phase to set a constant output for the first cycle of simulation.
      | 
      | <b>Sample Time</b>
      | Specify the sample time of the block, in seconds. Set to 0 to implement a continuous block.
      mask TypeOptions Freq: Power/Freq
      mask TypeOptions Vinit: Power/Vinit
      mask TypeOptions Iinit: Power/Iinit
      mask TypeOptions Ts: Power/Ts
  Power Factor1 : Display
  THD : powerlib_meascontrol/Measurements/THD  Freq=60  Ts=Ts_Power
      settings: SourceProductName=Simscape Electrical
  THD (% and signal) : Scope  NumInputPorts=2
  THD (%) : Display
      settings: Format=bank
  Vabc pu1 : Scope
  to % : Gain  Gain=100  SampleTime=Ts_Power
  wires:
  [Iabc_load_14] -> Power Factor Block1/2(Iabc)
  [Vabc_load_14] -> Power Factor Block1/1(Vabc), THD/1, THD (% and signal)/1  "Signal Vabc"
  THD/1 -> to %/1
  to %/1 -> THD (%)/1, THD (% and signal)/2  "THD (%)"
  Power Factor Block1/4(Iabc y Iabc (rms)) -> Measurement1/4
  Power Factor Block1/1(Pabc) -> Measurement1/1
  Conv pu1/1 -> Vabc pu1/1
  Power Factor Block1/5("PFabc ") -> Power Factor1/1
  Power Factor Block1/2(Qabc) -> Measurement1/2
  Power Factor Block1/3(Vabc y Vabc (rms)) -> Conv pu1/1, Measurement1/3

== system Model_14Bus_Microgrid_R2017b/Load_4 ==
  note: C
  note: B
  note: A
  note: C
  note: Linea - Neutro
  note: B
  note: A
  Conv pu1 : Gain  Gain=sqrt (3) /Vnom_prim  SaturateOnIntegerOverflow=on  OutDataTypeStr=Inherit: Same as input  ParamDataTypeStr=Inherit: Same as input
  Measurement1 : Scope  NumInputPorts=4
  Power Factor Block1 : Subsystem  mask(Power Factor Block){Freq=Fnom, Vinit=[0, 0], Iinit=[0, 0], Ts=0}
      mask prompts: Freq "Fundamental frequency (Hz):"; Vinit "Voltage initial input [ Mag, Phase (degrees) ]:"; Iinit "Current initial input [ Mag, Phase (degrees) ]:"; Ts "Sample time:"
      mask help:
      | Power Factor Block developed by Dr Rodney Tan
      | Version 1.01 (Aug 2016)
      |
      | Compute power factor and phase angle of AC circuit voltage-current pair at fundamental frequency.
      |
      | The computation is based on Power block and Complex number function block.
      |
      | For the first cycle of simulation, the outputs are held constant to the powers computed for the Voltage initial input and Current initial input parameters.
      mask Help:
      | <b>Fundamental Frequency (Hz)</b>
      | Specify the measurement fundamental frequency, in hertz, of the input signal.
      | 
      | <b>Voltage initial input [ Mag, Phase (degrees) ]</b>
      | Specify the voltage initial magnitude and phase to set a constant output for the first cycle of simulation.
      | 
      | <b>Current initial input [ Mag, Phase (degrees) ]</b>
      | Specify the current initial magnitude and phase to set a constant output for the first cycle of simulation.
      | 
      | <b>Sample Time</b>
      | Specify the sample time of the block, in seconds. Set to 0 to implement a continuous block.
      mask TypeOptions Freq: Power/Freq
      mask TypeOptions Vinit: Power/Vinit
      mask TypeOptions Iinit: Power/Iinit
      mask TypeOptions Ts: Power/Ts
  Power Factor1 : Display
  THD : powerlib_meascontrol/Measurements/THD  Freq=60  Ts=Ts_Power
      settings: SourceProductName=Simscape Electrical
  THD (% and signal) : Scope  NumInputPorts=2
  THD (%) : Display
      settings: Format=bank
  Vabc pu1 : Scope
  to % : Gain  Gain=100  SampleTime=Ts_Power
  wires:
  [Iabc_load_14_1] -> Power Factor Block1/2(Iabc)
  [Vabc_load_14_1] -> Power Factor Block1/1(Vabc), THD/1, THD (% and signal)/1  "Signal Vabc"
  THD/1 -> to %/1
  to %/1 -> THD (%)/1, THD (% and signal)/2  "THD (%)"
  Power Factor Block1/4(Iabc y Iabc (rms)) -> Measurement1/4
  Power Factor Block1/1(Pabc) -> Measurement1/1
  Conv pu1/1 -> Vabc pu1/1
  Power Factor Block1/5("PFabc ") -> Power Factor1/1
  Power Factor Block1/2(Qabc) -> Measurement1/2
  Power Factor Block1/3(Vabc y Vabc (rms)) -> Conv pu1/1, Measurement1/3

== system Model_14Bus_Microgrid_R2017b/Main Grid 69 kV Inf ==
  note: Thevenin equivalent
  69kV 100 MVA 1 : powerlib/Elements/Three-Phase Series RLC Branch  LConnTagsString=A|B|C  RConnTagsString=A|B|C  BranchType=RL  Resistance=69e3^2/100e6/10  Inductance=69e3^2/100e6/(2*pi*60)  Capacitance=1.0  Measurements=None
      settings: SourceProductName=Simscape Electrical
  Ground1 : powerlib/Elements/Ground  LConnTagsString=a
      settings: SourceProductName=Simscape Electrical
  Programmable Voltage Source1 : powerlib/Electrical Sources/Three-Phase Programmable Voltage Source  PositiveSequence="[69e3 0  60]"  VariationEntity=None  VariationType=Table of time-amplitude pairs  VariationTypeAlt=Step  VariationStep=-0.3  VariationRate=0.5  VariationMagnitude=0.4  VariationFrequency=2  VariationTiming=[0.1 1.2]  VariationPhaseA=off  Amplitudes=[1]  TimeValues=[0]  HarmonicGeneration=off  HarmonicA=[3 0.2 -25 0]  HarmonicB="[2 0.15  35 2]"  Timing="[0.1  0.6]"  BusType=swing  Pref=500  Qref=0  Qmin=-inf  Qmax=inf
      settings: SourceProductName=Simscape Electrical
  C : PMIOPort  Side=Right
  B : PMIOPort  Port=2  Side=Right
  A : PMIOPort  Port=3  Side=Right
  connections:
  Programmable Voltage Source1/RConn3 -- 69kV 100 MVA 1/LConn3
  Ground1/LConn1 -- Programmable Voltage Source1/LConn1
  Programmable Voltage Source1/RConn2 -- 69kV 100 MVA 1/LConn2
  69kV 100 MVA 1/LConn1 -- Programmable Voltage Source1/RConn1
  69kV 100 MVA 1/RConn3 -- C/RConn1
  69kV 100 MVA 1/RConn2 -- B/RConn1
  69kV 100 MVA 1/RConn1 -- A/RConn1
